simulink model "Test_Stand_Trans_Controller"  (R2022b)
settings: Solver=FixedStepAuto  StartTime=0.0  StopTime=3000  FixedStep=.01  RelTol=1e-3  EnableMultiTasking=on
libraries: canmsglib x4, raspberrypiCommlib x3
settings Model: Creator=david  LastModifiedBy=david
settings SolverCC: PositivePriorityOrder=on
settings OptimizationCC: EnhancedBackFolding=on  PassReuseOutputArgsAs=Individual arguments  ZeroExternalMemoryAtStartup=off  ZeroInternalMemoryAtStartup=off  MaxStackSize=64  OptimizeBlockOrder=speed  DifferentSizesBufferReuse=on  OptimizationCustomize=off  EfficientTunableParamExpr=on
settings DebuggingCC: ParameterTunabilityLossMsg=error
settings HardwareCC: ProdBitPerPointer=32  ProdBitPerSizeT=32  ProdBitPerPtrDiffT=32  ProdLargestAtomicInteger=Long  ProdLargestAtomicFloat=Double  ProdWordSize=32  ProdLongLongMode=on  ProdHWDeviceType=ARM Compatible->ARM Cortex
settings RTWCC: Description=Embedded Coder  SystemTargetFile=ert.tlc  HardwareBoard=Raspberry Pi  TLCOptions="-aInlineSetEventsForThisBaseRateFcn=TLC_FALSE -aSuppressMultiTaskScheduler=TLC_FALSE  -aRateBasedStepFcn=0"  TemplateMakefile=ert_default_tmf  Toolchain=GNU GCC Embedded Linux  BuildConfiguration=Faster Runs
settings CodeAppCC: ForceParamTrailComments=on  IgnoreCustomStorageClasses=off  OperatorAnnotations=on  SimulinkDataObjDesc=on  SFDataObjDesc=on  InsertBlockDesc=on
settings ERTTargetCC: SupportVariableSizeSignals=on  ExtModeTransport=2  ExtModeStaticAlloc=on  ExtModeMexFile=ext_xcp  ExtModeIntrfLevel=Level2 - Open

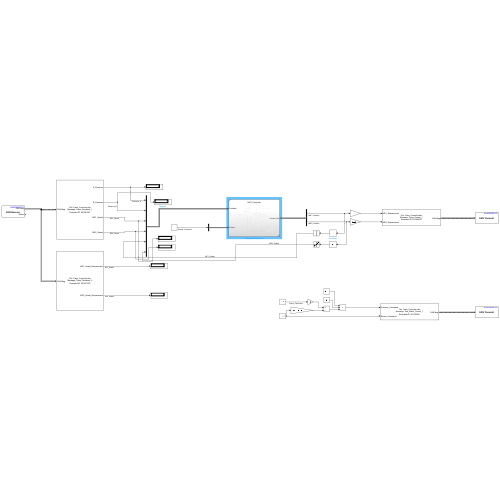
[thumbnail: Simulink's stored preview of the top-level diagram]
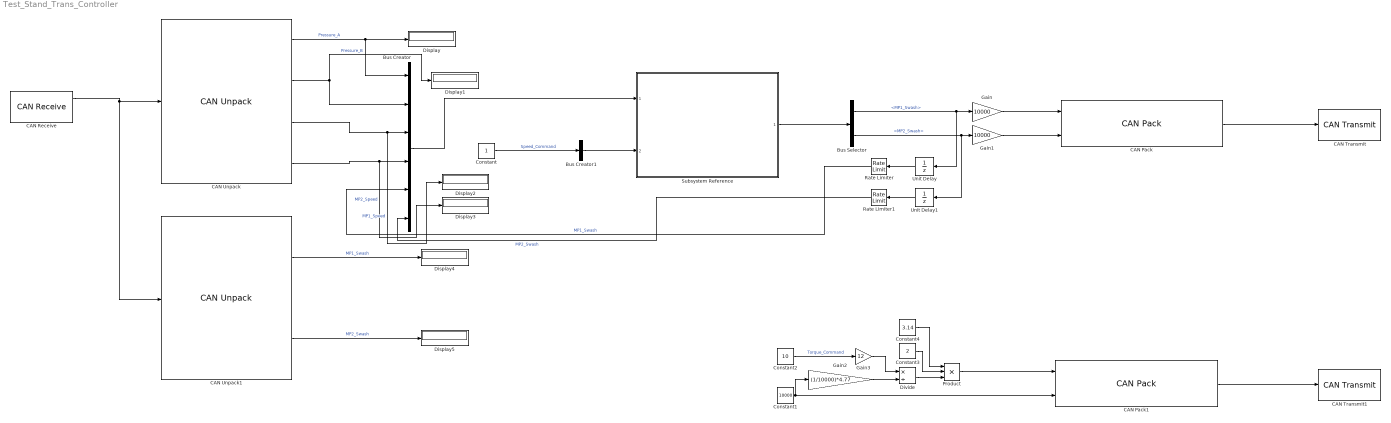
== system Test_Stand_Trans_Controller ==
  Bus Creator : BusCreator  Inputs=6
  Bus Creator1 : BusCreator  Inputs=1
  Bus Selector : BusSelector  OutputSignals=MP1_Swash,MP2_Swash
  CAN Pack : canmsglib/CAN Pack  CANdbFile=C:\Git\2023_Tractor_Plant_Models\23_Trans\Trans_Controller.dbc  MsgList=Trans_Control_1  MsgName=Trans_Control_1  MsgIDType=Extended (29-bit identifier)  MsgIdentifier=201392897  MsgLength=8  Remote=off  ApplyMinMax=off  BusOutput=on  SignalInfo={'MP1_Displacement','0','16','LE','unsigned','Standard','0','1','-10000','-10000','10000';'MP2_Displacement','16','16','LE','unsigned','Standard','0','1','-10000','-10000','10000'}
      settings: LibrarySourceBlock=embeddedtargetslib/Host Communication/CAN Pack  DataFormat=CANdb specified signals
  CAN Pack1 : canmsglib/CAN Pack  CANdbFile=C:\Git\2023_Tractor_Plant_Models\23_Trans\Trans_Controller.dbc  MsgList=Test_Stand_Control_1  MsgName=Test_Stand_Control_1  MsgIDType=Extended (29-bit identifier)  MsgIdentifier=201392641  MsgLength=8  Remote=off  ApplyMinMax=off  BusOutput=on  SignalInfo={'Pressure_Command','16','16','LE','unsigned','Standard','0','1','0','0','4000';'Swash_Command','0','16','LE','unsigned','Standard','0','1','-10000','-10000','10000'}
      settings: LibrarySourceBlock=embeddedtargetslib/Host Communication/CAN Pack  DataFormat=CANdb specified signals
  CAN Receive : raspberrypiCommlib/CAN Receive  DeviceID=can0  SetupCAN=off  TypeofCAN=Real  OutputDataType=CAN Msg  IdentifierType=Standard (11-bit identifier)  MessageId=100  MsgLength=8  SampleTime=-1  OutputError=off  OutputRemote=off  SimulateUsing=Code generation
  CAN Transmit : raspberrypiCommlib/CAN Transmit  DeviceID=can0  SetupCAN=on  TypeofCAN=Real  InputDataType=CAN Msg  BlockingMode_=off  BlockTimeout_=1  OutputStatus=off  IdentifierType=Standard (11-bit identifier)  MessageId=100  MsgLength=8  RemoteFrame=off  SimulateUsing=Code generation
  CAN Transmit1 : raspberrypiCommlib/CAN Transmit  DeviceID=can0  SetupCAN=off  TypeofCAN=Real  InputDataType=CAN Msg  BlockingMode_=off  BlockTimeout_=1  OutputStatus=off  IdentifierType=Standard (11-bit identifier)  MessageId=100  MsgLength=8  RemoteFrame=off  SimulateUsing=Code generation
  CAN Unpack : canmsglib/CAN Unpack  CANdbFile=C:\Git\2023_Tractor_Plant_Models\23_Trans\Trans_Controller.dbc  MsgList=Trans_Feedback_1  MsgName=Trans_Feedback_1  MsgIDType=Extended (29-bit identifier)  MsgIdentifier=201392387  MsgLength=8  SignalInfo={'A_Pressure','32','16','LE','unsigned','Standard','0','1','0','0','4500';'B_Pressure','48','16','LE','unsigned','Standard','0','1','0','0','4500';'MP1_Speed','0','16','LE','unsigned','Standard','0','1','0','0','4500';'MP2_Speed','16','16','LE','unsigned','Standard','0','1','0','0','4500'}  IDPort=off  TimestampPort=off  ErrorPort=off  RemotePort=off  LengthPort=off  StatusPort=off  ApplyMinMax=off
      settings: LibrarySourceBlock=embeddedtargetslib/Host Communication/CAN Unpack  DataFormat=CANdb specified signals
  CAN Unpack1 : canmsglib/CAN Unpack  CANdbFile=C:\Git\2023_Tractor_Plant_Models\23_Trans\Trans_Controller.dbc  MsgList=Trans_Feedback_2  MsgName=Trans_Feedback_2  MsgIDType=Extended (29-bit identifier)  MsgIdentifier=201457923  MsgLength=8  SignalInfo={'MP1_Actual_Displacement','0','16','LE','unsigned','Standard','0','1','-10000','-10000','10000';'MP2_Actual_Displacement','16','16','LE','unsigned','Standard','0','1','-10000','-10000','10000'}  IDPort=off  TimestampPort=off  ErrorPort=off  RemotePort=off  LengthPort=off  StatusPort=off  ApplyMinMax=off
      settings: LibrarySourceBlock=embeddedtargetslib/Host Communication/CAN Unpack  DataFormat=CANdb specified signals
  Constant : Constant
  Constant1 : Constant  Value=10000
  Constant2 : Constant  Value=10
  Constant3 : Constant  Value=2
  Constant4 : Constant  Value=3.14
  Display{,1..5} (6 alike) : Display
  Divide : Product  Inputs=*/
  Gain : Gain  Gain=10000
  Gain1 : Gain  Gain=10000
  Gain2 : Gain  Gain=(1/10000)*4.77
  Gain3 : Gain  Gain=12
  Product : Product  Inputs=3
  Rate Limiter : RateLimiter  RisingSlewLimit=.1  FallingSlewLimit=-.1  SampleTimeMode=inherited
  Rate Limiter1 : RateLimiter  RisingSlewLimit=.1  FallingSlewLimit=-.1  SampleTimeMode=inherited
  Subsystem Reference : Subsystem  ReferencedSubsystem=HMT_Controller
  Unit Delay : UnitDelay  SampleTime=-1  HasFrameUpgradeWarning=on
  Unit Delay1 : UnitDelay  SampleTime=-1  HasFrameUpgradeWarning=on
  wires:
  CAN Pack/1 -> CAN Transmit/1
  Subsystem Reference/1 -> Bus Selector/1
  Bus Selector/1 -> Unit Delay/1, Gain/1  "<MP1_Swash>"
  Bus Selector/2 -> Unit Delay1/1, Gain1/1  "<MP2_Swash>"
  Gain/1 -> CAN Pack/1
  Gain1/1 -> CAN Pack/2
  CAN Unpack/1 -> Display/1, Bus Creator/1  "Pressure_A"
  CAN Unpack/2 -> Display1/1, Bus Creator/2  "Pressure_B"
  Bus Creator/1 -> Subsystem Reference/1
  CAN Receive/1 -> CAN Unpack1/1, CAN Unpack/1
  Bus Creator1/1 -> Subsystem Reference/2
  Constant/1 -> Bus Creator1/1  "Speed_Command"
  CAN Unpack1/1 -> Display4/1  "MP1_Swash"
  CAN Unpack1/2 -> Display5/1  "MP2_Swash"
  CAN Unpack/4 -> Display3/1, Bus Creator/4  "MP2_Speed"
  CAN Unpack/3 -> Display2/1, Bus Creator/3  "MP1_Speed"
  CAN Pack1/1 -> CAN Transmit1/1
  Constant1/1 -> CAN Pack1/2, Gain2/1
  Gain2/1 -> Divide/2
  Constant2/1 -> Gain3/1  "Torque_Command"
  Divide/1 -> Product/3
  Constant4/1 -> Product/1
  Constant3/1 -> Product/2
  Product/1 -> CAN Pack1/1
  Gain3/1 -> Divide/1
  Unit Delay/1 -> Rate Limiter/1
  Unit Delay1/1 -> Rate Limiter1/1
  Rate Limiter/1 -> Bus Creator/5  "MP1_Swash"
  Rate Limiter1/1 -> Bus Creator/6  "MP2_Swash"
